simulink model "TST_ASDdc_Governor"  (R2016b)
settings: Solver=FixedStepDiscrete  StartTime=0.0  StopTime=simTime  FixedStep=sampleTime  RelTol=1e-3
values from neighbouring files (symbols this model uses):
  testCase = 1    [initTST_ASDdc_Governor_001.m]
libraries: simulink x3, UnitTest_Lib x1
settings Model: Creator=zhengjinyan  LastModifiedBy=zhengjinyan
settings DebuggingCC: SignalRangeChecking=error

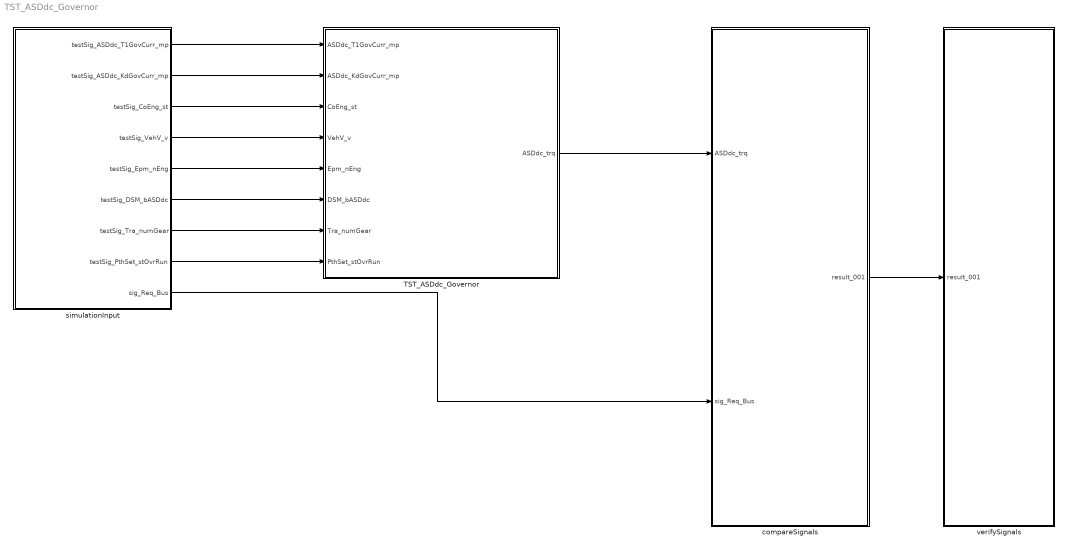
== system TST_ASDdc_Governor ==
  TST_ASDdc_Governor : Subsystem
  compareSignals : Subsystem
  simulationInput : Subsystem
  verifySignals : Subsystem
  wires:
  simulationInput/1(testSig_ASDdc_T1GovCurr_mp) -> TST_ASDdc_Governor/1(ASDdc_T1GovCurr_mp)
  simulationInput/2(testSig_ASDdc_KdGovCurr_mp) -> TST_ASDdc_Governor/2(ASDdc_KdGovCurr_mp)
  simulationInput/3(testSig_CoEng_st) -> TST_ASDdc_Governor/3(CoEng_st)
  simulationInput/4(testSig_VehV_v) -> TST_ASDdc_Governor/4(VehV_v)
  simulationInput/5(testSig_Epm_nEng) -> TST_ASDdc_Governor/5(Epm_nEng)
  simulationInput/6(testSig_DSM_bASDdc) -> TST_ASDdc_Governor/6(DSM_bASDdc)
  simulationInput/7(testSig_Tra_numGear) -> TST_ASDdc_Governor/7(Tra_numGear)
  simulationInput/8(testSig_PthSet_stOvrRun) -> TST_ASDdc_Governor/8(PthSet_stOvrRun)
  TST_ASDdc_Governor/1(ASDdc_trq) -> compareSignals/1(ASDdc_trq)
  simulationInput/9(sig_Req_Bus) -> compareSignals/2(sig_Req_Bus)
  compareSignals/1(result_001) -> verifySignals/1(result_001)

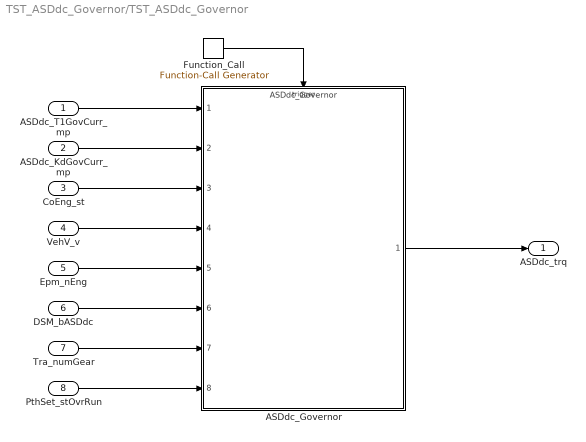
== system TST_ASDdc_Governor/TST_ASDdc_Governor ==
  ASDdc_T1GovCurr_mp : Inport
  ASDdc_KdGovCurr_mp : Inport  Port=2
  CoEng_st : Inport  Port=3
  VehV_v : Inport  Port=4
  Epm_nEng : Inport  Port=5
  DSM_bASDdc : Inport  Port=6
  Tra_numGear : Inport  Port=7
  PthSet_stOvrRun : Inport  Port=8
  ASDdc_Governor : ModelReference  ModelNameDialog=ASDdc_Governor  SimulationMode=Normal  ModelReferenceVersion=1.21  TriggerPortName=function  TriggerPortTriggerType=function-call  TriggerPortStatesWhenEnabling=held
  Function_Call : simulink/Ports & Subsystems/Function-Call Generator  sample_time=sampleTime  numberOfIterations=1
  ASDdc_trq : Outport
  wires:
  Function_Call/1 -> ASDdc_Governor/Trigger
  ASDdc_T1GovCurr_mp/1 -> ASDdc_Governor/1
  ASDdc_KdGovCurr_mp/1 -> ASDdc_Governor/2
  CoEng_st/1 -> ASDdc_Governor/3
  VehV_v/1 -> ASDdc_Governor/4
  Epm_nEng/1 -> ASDdc_Governor/5
  DSM_bASDdc/1 -> ASDdc_Governor/6
  Tra_numGear/1 -> ASDdc_Governor/7
  PthSet_stOvrRun/1 -> ASDdc_Governor/8
  ASDdc_Governor/1 -> ASDdc_trq/1

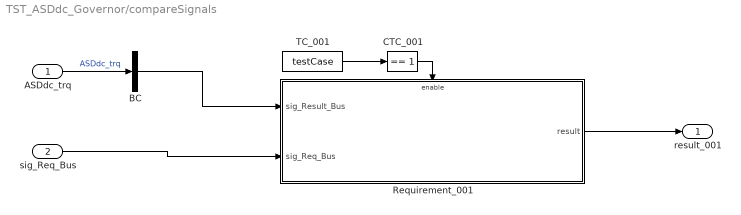
== system TST_ASDdc_Governor/compareSignals ==
  ASDdc_trq : Inport
  sig_Req_Bus : Inport  Port=2
  BC : BusCreator  Inputs=1
  CTC_001 : simulink/Logic and Bit Operations/Compare To Constant  relop===  const=1  OutDataTypeStr=boolean
  Requirement_001 : Subsystem
  TC_001 : Constant  Value=testCase
  result_001 : Outport
  wires:
  ASDdc_trq/1 -> BC/1  "ASDdc_trq"
  TC_001/1 -> CTC_001/1
  CTC_001/1 -> Requirement_001/Enable
  sig_Req_Bus/1 -> Requirement_001/2(sig_Req_Bus)
  BC/1 -> Requirement_001/1(sig_Result_Bus)
  Requirement_001/1(result) -> result_001/1

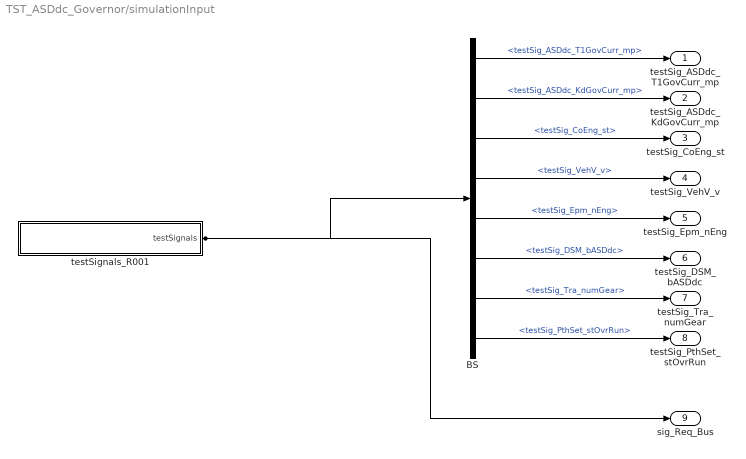
== system TST_ASDdc_Governor/simulationInput ==
  BS : BusSelector  OutputSignals=testSig_ASDdc_T1GovCurr_mp,testSig_ASDdc_KdGovCurr_mp,testSig_CoEng_st,testSig_VehV_v,testSig_Epm_nEng,testSig_DSM_bASDdc,testSig_Tra_numGear,testSig_PthSet_stOvrRun
  testSignals_R001 : Subsystem
  testSig_ASDdc_T1GovCurr_mp : Outport
  testSig_ASDdc_KdGovCurr_mp : Outport  Port=2
  testSig_CoEng_st : Outport  Port=3
  testSig_VehV_v : Outport  Port=4
  testSig_Epm_nEng : Outport  Port=5
  testSig_DSM_bASDdc : Outport  Port=6
  testSig_Tra_numGear : Outport  Port=7
  testSig_PthSet_stOvrRun : Outport  Port=8
  sig_Req_Bus : Outport  Port=9
  wires:
  BS/1 -> testSig_ASDdc_T1GovCurr_mp/1  "<testSig_ASDdc_T1GovCurr_mp>"
  BS/2 -> testSig_ASDdc_KdGovCurr_mp/1  "<testSig_ASDdc_KdGovCurr_mp>"
  BS/3 -> testSig_CoEng_st/1  "<testSig_CoEng_st>"
  BS/4 -> testSig_VehV_v/1  "<testSig_VehV_v>"
  BS/5 -> testSig_Epm_nEng/1  "<testSig_Epm_nEng>"
  BS/6 -> testSig_DSM_bASDdc/1  "<testSig_DSM_bASDdc>"
  BS/7 -> testSig_Tra_numGear/1  "<testSig_Tra_numGear>"
  BS/8 -> testSig_PthSet_stOvrRun/1  "<testSig_PthSet_stOvrRun>"
  testSignals_R001/1(testSignals) -> BS/1, sig_Req_Bus/1

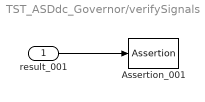
== system TST_ASDdc_Governor/verifySignals ==
  result_001 : Inport
  Assertion_001 : Assertion  Enabled=off
  wires:
  result_001/1 -> Assertion_001/1

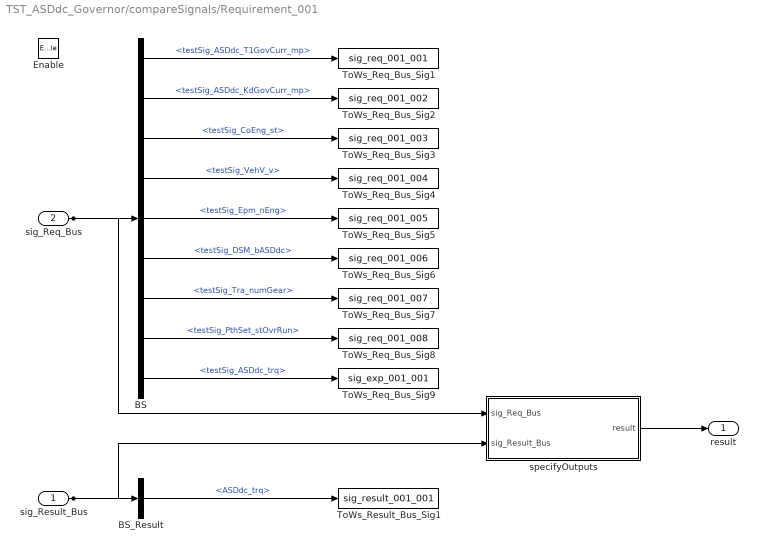
== system TST_ASDdc_Governor/compareSignals/Requirement_001 ==
  sig_Result_Bus : Inport
  sig_Req_Bus : Inport  Port=2
  Enable : EnablePort
  BS : BusSelector  OutputSignals=testSig_ASDdc_T1GovCurr_mp,testSig_ASDdc_KdGovCurr_mp,testSig_CoEng_st,testSig_VehV_v,testSig_Epm_nEng,testSig_DSM_bASDdc,testSig_Tra_numGear,testSig_PthSet_stOvrRun,testSig_ASDdc_trq
  BS_Result : BusSelector  OutputSignals=ASDdc_trq
  ToWs_Req_Bus_Sig1 : ToWorkspace  VariableName=sig_req_001_001  SaveFormat=Structure With Time
  ToWs_Req_Bus_Sig2 : ToWorkspace  VariableName=sig_req_001_002  SaveFormat=Structure With Time
  ToWs_Req_Bus_Sig3 : ToWorkspace  VariableName=sig_req_001_003  SaveFormat=Structure With Time
  ToWs_Req_Bus_Sig4 : ToWorkspace  VariableName=sig_req_001_004  SaveFormat=Structure With Time
  ToWs_Req_Bus_Sig5 : ToWorkspace  VariableName=sig_req_001_005  SaveFormat=Structure With Time
  ToWs_Req_Bus_Sig6 : ToWorkspace  VariableName=sig_req_001_006  SaveFormat=Structure With Time
  ToWs_Req_Bus_Sig7 : ToWorkspace  VariableName=sig_req_001_007  SaveFormat=Structure With Time
  ToWs_Req_Bus_Sig8 : ToWorkspace  VariableName=sig_req_001_008  SaveFormat=Structure With Time
  ToWs_Req_Bus_Sig9 : ToWorkspace  VariableName=sig_exp_001_001  SaveFormat=Structure With Time
  ToWs_Result_Bus_Sig1 : ToWorkspace  VariableName=sig_result_001_001  SaveFormat=Structure With Time
  specifyOutputs : Subsystem
  result : Outport
  wires:
  sig_Req_Bus/1 -> BS/1, specifyOutputs/1(sig_Req_Bus)
  BS/1 -> ToWs_Req_Bus_Sig1/1  "<testSig_ASDdc_T1GovCurr_mp>"
  BS/2 -> ToWs_Req_Bus_Sig2/1  "<testSig_ASDdc_KdGovCurr_mp>"
  BS/3 -> ToWs_Req_Bus_Sig3/1  "<testSig_CoEng_st>"
  BS/4 -> ToWs_Req_Bus_Sig4/1  "<testSig_VehV_v>"
  BS/5 -> ToWs_Req_Bus_Sig5/1  "<testSig_Epm_nEng>"
  BS/6 -> ToWs_Req_Bus_Sig6/1  "<testSig_DSM_bASDdc>"
  BS/7 -> ToWs_Req_Bus_Sig7/1  "<testSig_Tra_numGear>"
  BS/8 -> ToWs_Req_Bus_Sig8/1  "<testSig_PthSet_stOvrRun>"
  BS/9 -> ToWs_Req_Bus_Sig9/1  "<testSig_ASDdc_trq>"
  sig_Result_Bus/1 -> BS_Result/1, specifyOutputs/2(sig_Result_Bus)
  BS_Result/1 -> ToWs_Result_Bus_Sig1/1  "<ASDdc_trq>"
  specifyOutputs/1(result) -> result/1

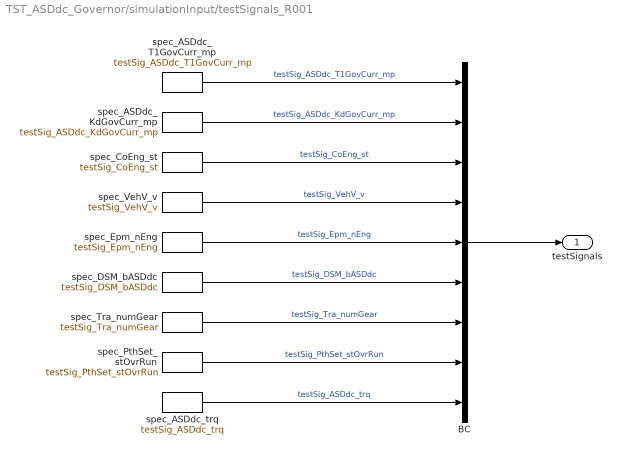
== system TST_ASDdc_Governor/simulationInput/testSignals_R001 ==
  BC : BusCreator  Inputs=9
  spec_ASDdc_KdGovCurr_mp : FromWorkspace  VariableName=testSig_ASDdc_KdGovCurr_mp  Interpolate=off  OutputAfterFinalValue=Holding final value
  spec_ASDdc_T1GovCurr_mp : FromWorkspace  VariableName=testSig_ASDdc_T1GovCurr_mp  Interpolate=off  OutputAfterFinalValue=Holding final value
  spec_ASDdc_trq : FromWorkspace  VariableName=testSig_ASDdc_trq  Interpolate=off  OutputAfterFinalValue=Holding final value
  spec_CoEng_st : FromWorkspace  VariableName=testSig_CoEng_st  Interpolate=off  OutputAfterFinalValue=Holding final value
  spec_DSM_bASDdc : FromWorkspace  VariableName=testSig_DSM_bASDdc  Interpolate=off  OutputAfterFinalValue=Holding final value
  spec_Epm_nEng : FromWorkspace  VariableName=testSig_Epm_nEng  Interpolate=off  OutputAfterFinalValue=Holding final value
  spec_PthSet_stOvrRun : FromWorkspace  VariableName=testSig_PthSet_stOvrRun  Interpolate=off  OutputAfterFinalValue=Holding final value
  spec_Tra_numGear : FromWorkspace  VariableName=testSig_Tra_numGear  Interpolate=off  OutputAfterFinalValue=Holding final value
  spec_VehV_v : FromWorkspace  VariableName=testSig_VehV_v  Interpolate=off  OutputAfterFinalValue=Holding final value
  testSignals : Outport
  wires:
  BC/1 -> testSignals/1
  spec_ASDdc_T1GovCurr_mp/1 -> BC/1  "testSig_ASDdc_T1GovCurr_mp"
  spec_ASDdc_KdGovCurr_mp/1 -> BC/2  "testSig_ASDdc_KdGovCurr_mp"
  spec_CoEng_st/1 -> BC/3  "testSig_CoEng_st"
  spec_VehV_v/1 -> BC/4  "testSig_VehV_v"
  spec_Epm_nEng/1 -> BC/5  "testSig_Epm_nEng"
  spec_DSM_bASDdc/1 -> BC/6  "testSig_DSM_bASDdc"
  spec_Tra_numGear/1 -> BC/7  "testSig_Tra_numGear"
  spec_PthSet_stOvrRun/1 -> BC/8  "testSig_PthSet_stOvrRun"
  spec_ASDdc_trq/1 -> BC/9  "testSig_ASDdc_trq"

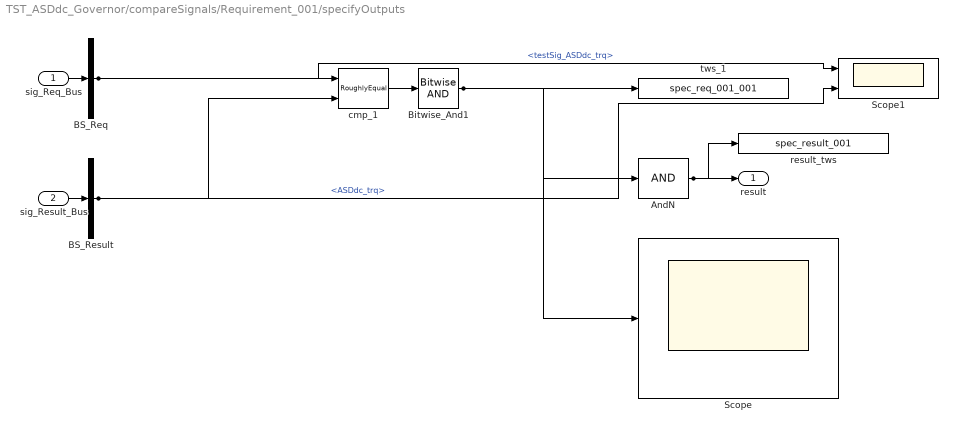
== system TST_ASDdc_Governor/compareSignals/Requirement_001/specifyOutputs ==
  sig_Req_Bus : Inport
  sig_Result_Bus : Inport  Port=2
  AndN : Logic  Inputs=1
  BS_Req : BusSelector  OutputSignals=testSig_ASDdc_trq
  BS_Result : BusSelector  OutputSignals=ASDdc_trq
  Bitwise_And1 : simulink/Logic and Bit Operations/Bitwise Operator  logicop=AND  UseBitMask=off  BitMask=bin2dec('11011001')  BitMaskRealWorld=Stored Integer
  Scope : Scope
  Scope1 : Scope  NumInputPorts=2
  cmp_1 : UnitTest_Lib/RoughlyEqual  slope=0.1
  result_tws : ToWorkspace  VariableName=spec_result_001
  tws_1 : ToWorkspace  VariableName=spec_req_001_001
  result : Outport
  wires:
  sig_Req_Bus/1 -> BS_Req/1
  sig_Result_Bus/1 -> BS_Result/1
  AndN/1 -> result/1, result_tws/1
  BS_Req/1 -> cmp_1/1, Scope1/1  "<testSig_ASDdc_trq>"
  BS_Result/1 -> cmp_1/2, Scope1/2  "<ASDdc_trq>"
  cmp_1/1 -> Bitwise_And1/1
  Bitwise_And1/1 -> tws_1/1, AndN/1, Scope/1
